simulink library "chassisLibrary"  (R2022b)
settings: Solver=VariableStepAuto  StartTime=0.0  StopTime=10.0  RelTol=1e-3
undefined symbols (not defined in the file): chassis
libraries: wheelLibrary x1
settings Model: Creator=ericb  LastModifiedBy=ericb
settings SolverCC: AlgebraicLoopSolver=TrustRegion
settings DebuggingCC: UnconnectedInputMsg=warning  UnconnectedOutputMsg=warning  UnconnectedLineMsg=warning  SFMachineParentedDataDiag=warning
settings ModelReferenceCC: EnableRefExpFcnMdlSchedulingChecks=on
settings RTWCC: DLArmComputeVersion=19.05

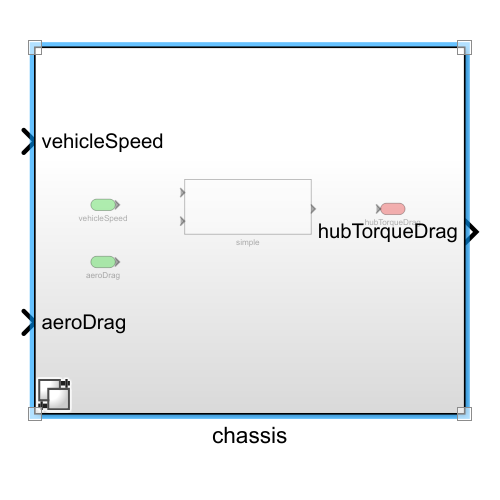
[thumbnail: Simulink's stored preview of the top-level diagram]
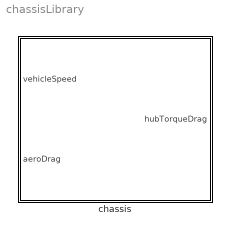
== system chassisLibrary ==
  chassis : Subsystem  Variant=on  PropagateVariantConditions=on

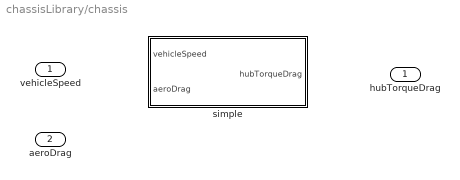
== system chassisLibrary/chassis ==
  vehicleSpeed : Inport
  aeroDrag : Inport  Port=2
  simple : Subsystem  VariantControl=strcmp(chassis.blockChoice, 'simple')
  hubTorqueDrag : Outport

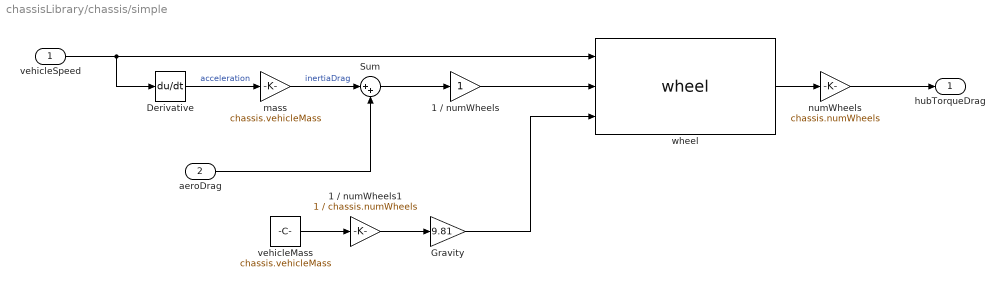
== system chassisLibrary/chassis/simple ==
  vehicleSpeed : Inport
  aeroDrag : Inport  Port=2
  1 / numWheels : Gain
  1 / numWheels1 : Gain  Gain=1 / chassis.numWheels
  Derivative : Derivative
  Gravity : Gain  Gain=9.81
  Sum : Sum  Inputs=|++
  mass : Gain  Gain=chassis.vehicleMass
  numWheels : Gain  Gain=chassis.numWheels
  vehicleMass : Constant  Value=chassis.vehicleMass
  wheel : wheelLibrary/wheel  SystemSampleTime=-1  VariantActivationTime=update diagram  Latency=0  AutoFrameSizeCalculation=off
  hubTorqueDrag : Outport
  wires:
  vehicleSpeed/1 -> Derivative/1, wheel/1
  Derivative/1 -> mass/1  "acceleration"
  mass/1 -> Sum/1  "inertiaDrag"
  aeroDrag/1 -> Sum/2
  wheel/1 -> numWheels/1
  numWheels/1 -> hubTorqueDrag/1
  Gravity/1 -> wheel/3
  vehicleMass/1 -> 1 / numWheels1/1
  1 / numWheels1/1 -> Gravity/1
  Sum/1 -> 1 / numWheels/1
  1 / numWheels/1 -> wheel/2
